simulink model "barebones_roll_pitch_model"  (R2021a)
settings: Solver=VariableStepAuto  StartTime=0.0  StopTime=100  RelTol=1e-3
undefined symbols (not defined in the file): J0, J1, Kt0, Kt1, Kv0, Kv1, mu_coulomb0, mu_coulomb1, mu_viscous0, mu_viscous1, ratio0, ratio1, v00, v01
libraries: simulink_extras x2, pid_lib x2
settings Model: Creator=ascalzo  LastModifiedBy=mfussi

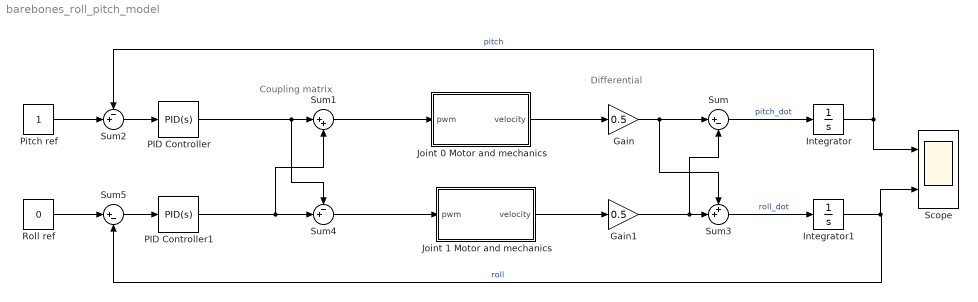
== system barebones_roll_pitch_model ==
  note: Coupling matrix
  note: Differential
  Gain : Gain  Gain=0.5
  Gain1 : Gain  Gain=0.5
  Integrator : Integrator
  Integrator1 : Integrator
  Joint 0 Motor and mechanics : Subsystem
  Joint 1 Motor and mechanics : Subsystem
  PID Controller : pid_lib/PID Controller  Controller=PID  Form=Parallel  TimeDomain=Continuous-time  UseExternalTs=off  SampleTime=-1  IntegratorMethod=Forward Euler  FilterMethod=Forward Euler  ControllerParametersSource=internal  P=10  I=5  D=0  UseFilter=on  N=100  TunerSelectOption=Transfer Function Based (PID Tuner App)  InitialConditionSource=internal  InitialConditionForIntegrator=0  InitialConditionForFilter=0  DifferentiatorICPrevScaledInput=0  ExternalReset=none  TrackingMode=off  Kt=1  LimitOutput=off  SatLimitsSource=internal  UpperSaturationLimit=inf  LowerSaturationLimit=-inf  LinearizeAsGain=on  AntiWindupMode=none  Kb=1  POutMin=[]  POutMax=[]  IOutMin=[]  IOutMax=[]  DOutMin=[]  DOutMax=[]  NOutMin=[]  NOutMax=[]  SumOutMin=[]  SumOutMax=[]  SaturationOutMin=[]  SaturationOutMax=[]  PParamMin=[]  PParamMax=[]  IParamMin=[]  IParamMax=[]  DParamMin=[]  DParamMax=[]  NParamMin=[]  NParamMax=[]  KbParamMin=[]  KbParamMax=[]  KtParamMin=[]  KtParamMax=[]  KbOutMin=[]  KbOutMax=[]  KtOutMin=[]  KtOutMax=[]  IntegratorOutMin=[]  IntegratorOutMax=[]  FilterOutMin=[]  FilterOutMax=[]  SumI1OutMin=[]  SumI1OutMax=[]  SumI2OutMin=[]  SumI2OutMax=[]  SumI3OutMin=[]  SumI3OutMax=[]  SumI4OutMin=[]  SumI4OutMax=[]  SumDOutMin=[]  SumDOutMax=[]  DifferentiatorOutMin=[]  DifferentiatorOutMax=[]  FilterDiffOutCoefMin=[]  FilterDiffOutCoefMax=[]  ReciprocalOutMin=[]  ReciprocalOutMax=[]  SumDenOutMin=[]  SumDenOutMax=[]  SumNumOutMin=[]  SumNumOutMax=[]  DivideOutMin=[]  DivideOutMax=[]  UdiffTsProdOutMin=[]  UdiffTsProdOutMax=[]  NTsProdOutMin=[]  NTsProdOutMax=[]  UintegralTsProdOutMin=[]  UintegralTsProdOutMax=[]  UngainTsProdOutMin=[]  UngainTsProdOutMax=[]  IntegratorContinuousStateAttributes=''  IntegratorStateMustResolveToSignalObject=off  IntegratorRTWStateStorageClass=Auto  FilterContinuousStateAttributes=''  FilterStateMustResolveToSignalObject=off  FilterRTWStateStorageClass=Auto  ParallelPVariant=InternalParameters  IdealPVariant=Disabled  IVariant=InternalParameters  DVariant=InternalParameters  IntegratorVariant=Continuous  SatVariant=Disabled  AWVariant=Passthrough  PCopyVariant=Disabled  TRVariant=Disabled  FdbkBlocksVariant=Forward  IdealPFdbkVariant=Disabled  SatFdbkVariant=Disabled  DerivativeFilterVariant=ContFilter  NVariant=InternalParameters  NCopyVariant=Disabled  FilterICVariant=InternalICsFilter  IntegratorICVariant=InternalICs  ExternalResetVariant=Disabled  TRSumVariant=Passthrough  SumFdbkVariant=Disabled  SumVariant=Sum_PID  TsampFilterVariant=InternalTs  TsampNgainVariant=Passthrough  TsampIntegralVariant=Passthrough  ExternalSaturationOutDataTypeStr=Inherit: Same as second input
  PID Controller1 : pid_lib/PID Controller  Controller=PID  Form=Parallel  TimeDomain=Continuous-time  UseExternalTs=off  SampleTime=-1  IntegratorMethod=Forward Euler  FilterMethod=Forward Euler  ControllerParametersSource=internal  P=10  I=5  D=0  UseFilter=on  N=100  TunerSelectOption=Transfer Function Based (PID Tuner App)  InitialConditionSource=internal  InitialConditionForIntegrator=0  InitialConditionForFilter=0  DifferentiatorICPrevScaledInput=0  ExternalReset=none  TrackingMode=off  Kt=1  LimitOutput=off  SatLimitsSource=internal  UpperSaturationLimit=inf  LowerSaturationLimit=-inf  LinearizeAsGain=on  AntiWindupMode=none  Kb=1  POutMin=[]  POutMax=[]  IOutMin=[]  IOutMax=[]  DOutMin=[]  DOutMax=[]  NOutMin=[]  NOutMax=[]  SumOutMin=[]  SumOutMax=[]  SaturationOutMin=[]  SaturationOutMax=[]  PParamMin=[]  PParamMax=[]  IParamMin=[]  IParamMax=[]  DParamMin=[]  DParamMax=[]  NParamMin=[]  NParamMax=[]  KbParamMin=[]  KbParamMax=[]  KtParamMin=[]  KtParamMax=[]  KbOutMin=[]  KbOutMax=[]  KtOutMin=[]  KtOutMax=[]  IntegratorOutMin=[]  IntegratorOutMax=[]  FilterOutMin=[]  FilterOutMax=[]  SumI1OutMin=[]  SumI1OutMax=[]  SumI2OutMin=[]  SumI2OutMax=[]  SumI3OutMin=[]  SumI3OutMax=[]  SumI4OutMin=[]  SumI4OutMax=[]  SumDOutMin=[]  SumDOutMax=[]  DifferentiatorOutMin=[]  DifferentiatorOutMax=[]  FilterDiffOutCoefMin=[]  FilterDiffOutCoefMax=[]  ReciprocalOutMin=[]  ReciprocalOutMax=[]  SumDenOutMin=[]  SumDenOutMax=[]  SumNumOutMin=[]  SumNumOutMax=[]  DivideOutMin=[]  DivideOutMax=[]  UdiffTsProdOutMin=[]  UdiffTsProdOutMax=[]  NTsProdOutMin=[]  NTsProdOutMax=[]  UintegralTsProdOutMin=[]  UintegralTsProdOutMax=[]  UngainTsProdOutMin=[]  UngainTsProdOutMax=[]  IntegratorContinuousStateAttributes=''  IntegratorStateMustResolveToSignalObject=off  IntegratorRTWStateStorageClass=Auto  FilterContinuousStateAttributes=''  FilterStateMustResolveToSignalObject=off  FilterRTWStateStorageClass=Auto  ParallelPVariant=InternalParameters  IdealPVariant=Disabled  IVariant=InternalParameters  DVariant=InternalParameters  IntegratorVariant=Continuous  SatVariant=Disabled  AWVariant=Passthrough  PCopyVariant=Disabled  TRVariant=Disabled  FdbkBlocksVariant=Forward  IdealPFdbkVariant=Disabled  SatFdbkVariant=Disabled  DerivativeFilterVariant=ContFilter  NVariant=InternalParameters  NCopyVariant=Disabled  FilterICVariant=InternalICsFilter  IntegratorICVariant=InternalICs  ExternalResetVariant=Disabled  TRSumVariant=Passthrough  SumFdbkVariant=Disabled  SumVariant=Sum_PID  TsampFilterVariant=InternalTs  TsampNgainVariant=Passthrough  TsampIntegralVariant=Passthrough  ExternalSaturationOutDataTypeStr=Inherit: Same as second input
  Pitch ref : Constant
  Roll ref : Constant  Value=0
  Scope : Scope  NumInputPorts=2
  Sum : Sum  Inputs=|+-
  Sum1 : Sum  Inputs=|++
  Sum2 : Sum  Inputs=-+|
  Sum3 : Sum  Inputs=++|
  Sum4 : Sum  Inputs=-+|
  Sum5 : Sum  Inputs=|+-
  wires:
  Joint 0 Motor and mechanics/1(velocity) -> Gain/1
  Sum1/1 -> Joint 0 Motor and mechanics/1(pwm)
  Sum2/1 -> PID Controller/1
  Sum/1 -> Integrator/1  "pitch_dot"
  Pitch ref/1 -> Sum2/2
  Sum5/1 -> PID Controller1/1
  PID Controller1/1 -> Sum4/2, Sum1/2
  Joint 1 Motor and mechanics/1(velocity) -> Gain1/1
  Sum4/1 -> Joint 1 Motor and mechanics/1(pwm)
  Sum3/1 -> Integrator1/1  "roll_dot"
  Roll ref/1 -> Sum5/1
  Gain/1 -> Sum/1, Sum3/1
  Gain1/1 -> Sum/2, Sum3/2
  PID Controller/1 -> Sum4/1, Sum1/1
  Integrator/1 -> Scope/1, Sum2/1  "pitch"
  Integrator1/1 -> Scope/2, Sum5/2  "roll"

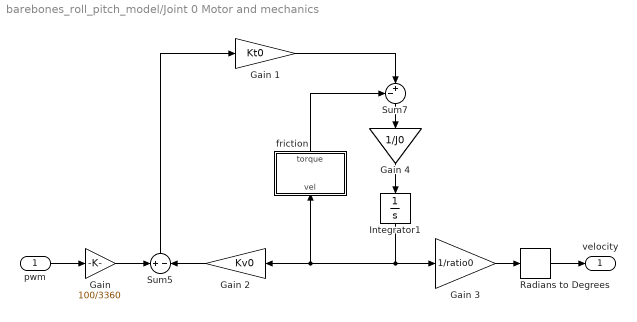
== system barebones_roll_pitch_model/Joint 0 Motor and mechanics ==
  pwm : Inport
  Gain : Gain  Gain=100/3360
  Gain 1 : Gain  Gain=Kt0
  Gain 2 : Gain  Gain=Kv0
  Gain 3 : Gain  Gain=1/ratio0
  Gain 4 : Gain  Gain=1/J0
  Integrator1 : Integrator  InitialCondition=v00*pi/180
  Radians to Degrees : simulink_extras/Transformations/Radians to Degrees
  Sum5 : Sum  Inputs=+|-
  Sum7 : Sum  Inputs=-+|
  friction : Subsystem
      mask Display: disp('differentiable\nfriction');
  velocity : Outport
  wires:
  Gain 2/1 -> Sum5/2
  Integrator1/1 -> Gain 2/1, friction/1(vel), Gain 3/1
  friction/1(torque) -> Sum7/1
  Gain 1/1 -> Sum7/2
  Sum5/1 -> Gain 1/1
  Sum7/1 -> Gain 4/1
  Gain 3/1 -> Radians to Degrees/1
  pwm/1 -> Gain/1
  Gain 4/1 -> Integrator1/1
  Radians to Degrees/1 -> velocity/1
  Gain/1 -> Sum5/1

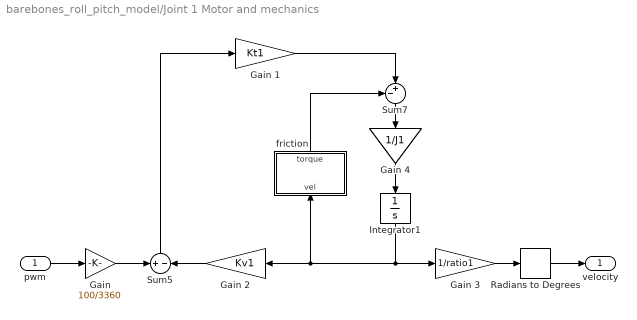
== system barebones_roll_pitch_model/Joint 1 Motor and mechanics ==
  pwm : Inport
  Gain : Gain  Gain=100/3360
  Gain 1 : Gain  Gain=Kt1
  Gain 2 : Gain  Gain=Kv1
  Gain 3 : Gain  Gain=1/ratio1
  Gain 4 : Gain  Gain=1/J1
  Integrator1 : Integrator  InitialCondition=v01*pi/180
  Radians to Degrees : simulink_extras/Transformations/Radians to Degrees
  Sum5 : Sum  Inputs=+|-
  Sum7 : Sum  Inputs=-+|
  friction : Subsystem
      mask Display: disp('differentiable\nfriction');
  velocity : Outport
  wires:
  Gain 2/1 -> Sum5/2
  Integrator1/1 -> Gain 2/1, friction/1(vel), Gain 3/1
  friction/1(torque) -> Sum7/1
  Gain 1/1 -> Sum7/2
  Sum5/1 -> Gain 1/1
  Sum7/1 -> Gain 4/1
  Gain 3/1 -> Radians to Degrees/1
  pwm/1 -> Gain/1
  Gain 4/1 -> Integrator1/1
  Radians to Degrees/1 -> velocity/1
  Gain/1 -> Sum5/1

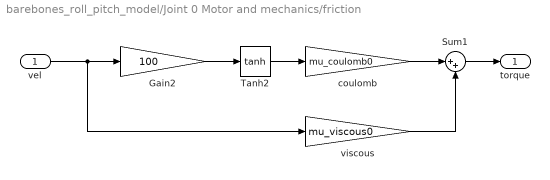
== system barebones_roll_pitch_model/Joint 0 Motor and mechanics/friction ==
  vel : Inport
  Gain2 : Gain  Gain=100
  Sum1 : Sum  Inputs=|++
  Tanh2 : Trigonometry  Operator=tanh
  coulomb : Gain  Gain=mu_coulomb0
  viscous : Gain  Gain=mu_viscous0
  torque : Outport
  wires:
  vel/1 -> viscous/1, Gain2/1
  Gain2/1 -> Tanh2/1
  Tanh2/1 -> coulomb/1
  Sum1/1 -> torque/1
  coulomb/1 -> Sum1/1
  viscous/1 -> Sum1/2

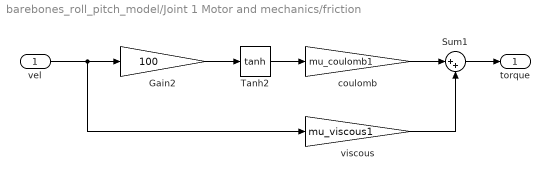
== system barebones_roll_pitch_model/Joint 1 Motor and mechanics/friction ==
  vel : Inport
  Gain2 : Gain  Gain=100
  Sum1 : Sum  Inputs=|++
  Tanh2 : Trigonometry  Operator=tanh
  coulomb : Gain  Gain=mu_coulomb1
  viscous : Gain  Gain=mu_viscous1
  torque : Outport
  wires:
  vel/1 -> viscous/1, Gain2/1
  Gain2/1 -> Tanh2/1
  Tanh2/1 -> coulomb/1
  Sum1/1 -> torque/1
  coulomb/1 -> Sum1/1
  viscous/1 -> Sum1/2
